simulink model "sampleModel1449_2_sub_sub"  (R2023a)
settings: Solver=VariableStepAuto  StartTime=0.0  StopTime=10.0  RelTol=1e-3
libraries: hdlsllib x6, simulink x1
settings Model: Creator=user1  LastModifiedBy=user1

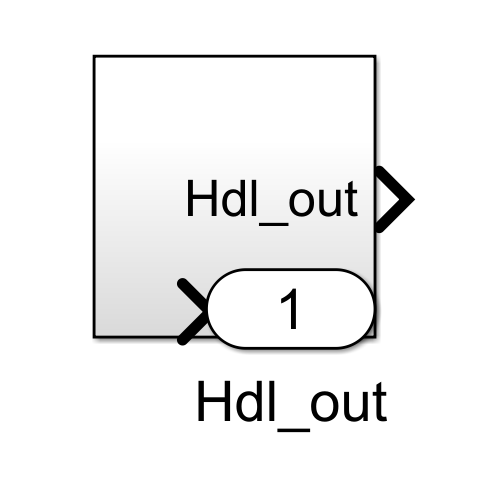
[thumbnail: Simulink's stored preview of the top-level diagram]
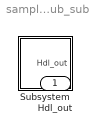
== system sampleModel1449_2_sub_sub ==
  Subsystem : Subsystem
  Hdl_out : Outport  OutDataTypeStr=uint8

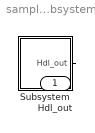
== system sampleModel1449_2_sub_sub/Subsystem ==
  Subsystem : Subsystem
  Hdl_out : Outport  OutDataTypeStr=uint8
  wires:
  Subsystem/1(Hdl_out) -> Hdl_out/1

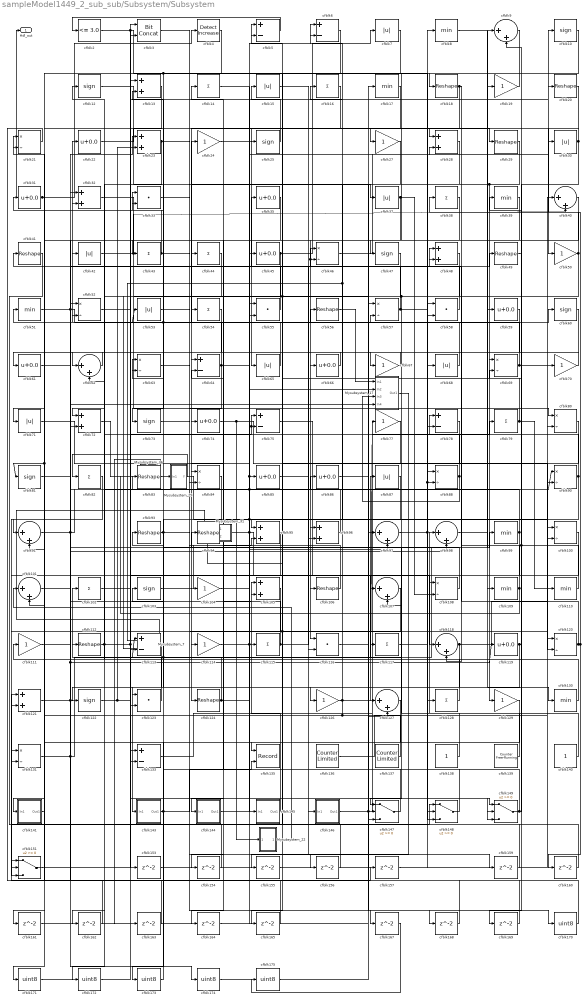
== system sampleModel1449_2_sub_sub/Subsystem/Subsystem ==
  Mysubsystem_17 : Subsystem  TreatAsAtomicUnit=on  RTWFcnName=Mysubsystem_17
      settings: RTWFcnNameOpts=User specified  RTWFileNameOpts=Use function name
  Mysubsystem_22 : Subsystem  TreatAsAtomicUnit=on  RTWFcnName=Mysubsystem_22
      settings: RTWFcnNameOpts=User specified  RTWFileNameOpts=Use function name
  Mysubsystem_29 : Subsystem  TreatAsAtomicUnit=on  RTWFcnName=Mysubsystem_29
      settings: RTWFcnNameOpts=User specified  RTWFileNameOpts=Use function name
  Mysubsystem_31 : Subsystem  TreatAsAtomicUnit=on  RTWFcnName=Mysubsystem_31
      settings: RTWFcnNameOpts=User specified  RTWFileNameOpts=Use function name
  Mysubsystem_36 : Subsystem  TreatAsAtomicUnit=on  RTWFcnName=Mysubsystem_36
      settings: RTWFcnNameOpts=User specified  RTWFileNameOpts=Use function name
  Mysubsystem_7 : Subsystem  TreatAsAtomicUnit=on  RTWFcnName=Mysubsystem_7
      settings: RTWFcnNameOpts=User specified  RTWFileNameOpts=Use function name
  cfblk{10,12,25,47,60,73,81,103,122} (9 alike) : Signum
  cfblk{21,46,52,57,63,69,80,84,88,90,100,108,120,131} (14 alike) : Product  Inputs=*/  OutDataTypeStr=uint8  RndMeth=Zero  SaturateOnIntegerOverflow=on
  cfblk{9,40,62,91,97..98,101,107,118,127} (10 alike) : Sum  Inputs=|++  OutDataTypeStr=uint8
  cfblk{14,16,38,43..44,54,79,82,102,115,117,128} (12 alike) : Sum  Inputs=+  OutDataTypeStr=uint8
  cfblk{19,24,27,50,67,70,77,104,111,114,126,129} (12 alike) : Gain  OutDataTypeStr=uint8
  cfblk{13,23,28,32,48,72,95..96,105,121} (10 alike) : Sum  OutDataTypeStr=uint8
  cfblk{18,20,29,41,49,56,83,93..94,106,112,124} (12 alike) : Reshape
  cfblk{8,17,39,51,99,109..110,130} (8 alike) : MinMax  OutDataTypeStr=uint8
  cfblk{5..6,64,75,78,113,133} (7 alike) : Sum  Inputs=+-  OutDataTypeStr=uint8
  cfblk{33,55,58,116,123} (5 alike) : DotProduct  OutDataTypeStr=uint8
  cfblk{22,31,35,45,59,61,66,74,85..86,119} (11 alike) : Bias  Bias=0.0  SaturateOnIntegerOverflow=off
  cfblk135 : Record  FileSettingsInternal="{\"entries\":[{\"content\":{\"excelSettings\":{\"content\":{},\"type\":\"Streamout.ExcelSettings\"}},\"type\":\"Streamout.FileSettingStorage\",\"uuid\":\"\"}],\"packageUris\":[\"http:\\/\\/schema.mathworks.com\\/mf0\\/streamout_blocks\\/R2020a\"],\"version\":\"1.0\"}"  Layout=[1 1]  SignalsInternal="{\"entries\":[{\"content\":{\"signals\":[{\"content\":{\"blockPath\":[],\"dimensions\":[1],\"domain\":\"\",\"lineColor\":\"#a2142f\",\"plots\":[1],\"port\":1,\"signalID\":18032,\"signalName\":\"cfblk48\"},\"type\":\"RecordBlkView.Signal\",\"uuid\":\"\"},{\"content\":{\"blockPath\":[],\"dimensions\":[1],\"domain\":\"\",\"lineColor\":\"#139fff\",\"plots\":[1],\"port\":2,\"signalID\":18035,\"signalName\":\"cfblk143\"},\"type\":\"RecordBlkView.Signal\",\"uuid\":\"\"}]},\"type\":\"RecordBlkView.InputSignals\",\"uuid\":\"\"}],\"packageUris\":[\"http:\\/\\/schema.mathworks.com\\/mf0\\/streamout_blocks\\/R2020a\"],\"version\":\"1.0\"}"  VisualizationBindings="{\"xyplotplugin\":{\"info\":[{\"series\":[{\"bindingParametersList\":[{\"parameter\":\"X-Axis\",\"signalID\":18032,\"signalName\":\"cfblk48\"},{\"parameter\":\"Y-Axis\",\"signalID\":18035,\"signalName\":\"cfblk143\"}],\"seriesID\":15856}],\"subplotID\":1}]}}"  CompatibilityTag=XY  st=-1
  cfblk136 : hdlsllib/Sources/Counter Limited  uplimit=7  tsamp=-1
  cfblk137 : hdlsllib/Sources/Counter Limited  uplimit=7  tsamp=-1
  cfblk138 : Constant  OutDataTypeStr=uint8  SampleTime=-1
  cfblk139 : hdlsllib/Sources/Counter Free-Running  NumBits=16  tsamp=-1
  cfblk140 : Constant  OutDataTypeStr=uint8  SampleTime=-1
  cfblk141 : Subsystem
      settings: LibrarySourceBlock=|
      | hdlsllib/Ports &
      | Subsystems/Subsystem
  cfblk143 : Subsystem
      settings: LibrarySourceBlock=|
      | hdlsllib/Ports &
      | Subsystems/Subsystem
  cfblk144 : Subsystem
      settings: LibrarySourceBlock=|
      | hdlsllib/Ports &
      | Subsystems/Subsystem
  cfblk145 : Subsystem
      settings: LibrarySourceBlock=|
      | hdlsllib/Ports &
      | Subsystems/Subsystem
  cfblk146 : Subsystem
      settings: LibrarySourceBlock=|
      | hdlsllib/Ports &
      | Subsystems/Subsystem
  cfblk{147..149,151} (4 alike) : Switch  OutDataTypeStr=uint8  SaturateOnIntegerOverflow=off  InputSameDT=off
  cfblk{7,15,30,37,42,53,65,68,71,87} (10 alike) : Abs  OutDataTypeStr=uint8  SaturateOnIntegerOverflow=off
  cfblk{153..157,159..165,167..169} (15 alike) : Delay  SampleTime=1
  cfblk{170..175} (6 alike) : DataTypeConversion  OutDataTypeStr=uint8  SaturateOnIntegerOverflow=off  RndMeth=Floor
  cfblk2 : hdlsllib/Logic and Bit Operations/Compare To Constant  relop=<=  const=3.0  OutDataTypeStr=uint8
  cfblk3 : hdlsllib/Logic and Bit Operations/Bit Concat  numInputs=2
  cfblk4 : simulink/Logic and Bit Operations/Detect Increase  vinit=0.0  OutDataTypeStr=uint8
      settings: LibrarySourceBlock=|
      | hdlsllib/Logic and Bit
      | Operations/Detect
      | Increase
  Hdl_out : Outport  OutDataTypeStr=uint8
  wires:
  Mysubsystem_36/1(Out1) -> cfblk163/1
  cfblk72/1 -> Mysubsystem_36/1(In1)
  Mysubsystem_7/1(Out1) -> Mysubsystem_31/2(In2)
  Mysubsystem_29/1(Y) -> cfblk82/1
  Mysubsystem_22/1(Out1) -> cfblk101/1
  Mysubsystem_17/1(Out1) -> cfblk155/1
  cfblk56/1 -> Mysubsystem_17/1(In1)
  cfblk175/1 -> cfblk127/2
  cfblk167/1 -> cfblk175/1
  cfblk174/1 -> cfblk127/1
  cfblk173/1 -> cfblk103/1
  cfblk127/1 -> cfblk173/1
  cfblk172/1 -> cfblk3/2
  cfblk171/1 -> cfblk3/1
  cfblk129/1 -> cfblk171/1
  cfblk170/1 -> cfblk52/1
  cfblk3/1 -> cfblk170/1
  cfblk169/1 -> cfblk151/2
  cfblk49/1 -> cfblk169/1
  cfblk168/1 -> cfblk121/1
  cfblk86/1 -> cfblk168/1
  cfblk165/1 -> cfblk133/1
  cfblk9/1 -> cfblk165/1
  cfblk164/1 -> cfblk57/1
  cfblk39/1 -> cfblk164/1
  cfblk163/1 -> cfblk91/2
  cfblk162/1 -> cfblk151/1
  cfblk161/1 -> cfblk55/1
  cfblk160/1 -> cfblk5/2
  cfblk159/1 -> cfblk131/1
  cfblk15/1 -> cfblk159/1
  cfblk157/1 -> cfblk100/1
  cfblk21/1 -> cfblk157/1
  cfblk156/1 -> cfblk13/1
  cfblk63/1 -> cfblk156/1
  cfblk155/1 -> cfblk88/1
  cfblk154/1 -> cfblk32/1
  cfblk95/1 -> cfblk154/1
  cfblk153/1 -> cfblk58/2
  cfblk102/1 -> cfblk153/1
  cfblk7/1 -> cfblk101/2, cfblk43/1
  cfblk77/1 -> cfblk96/2
  cfblk148/1 -> cfblk64/2
  cfblk94/1 -> cfblk148/3, cfblk120/2
  cfblk105/1 -> cfblk131/2
  cfblk81/1 -> cfblk23/1
  cfblk136/1 -> cfblk70/1
  cfblk54/1 -> cfblk91/1
  cfblk80/1 -> cfblk148/2
  cfblk65/1 -> cfblk21/1
  cfblk90/1 -> cfblk107/2, cfblk32/2
  cfblk118/1 -> cfblk122/1, cfblk80/2
  cfblk10/1 -> cfblk47/1
  cfblk146/1(Out1) -> cfblk68/1, cfblk149/2
  cfblk30/1 -> cfblk69/1, cfblk28/1
  cfblk53/1 -> cfblk57/2
  cfblk66/1 -> cfblk64/1
  cfblk33/1 -> cfblk78/2
  cfblk69/1 -> cfblk40/1, cfblk42/1
  cfblk103/1 -> cfblk55/2
  cfblk27/1 -> cfblk96/1
  cfblk70/1 -> cfblk67/1
  cfblk122/1 -> cfblk20/1, cfblk23/2
  cfblk79/1 -> cfblk5/1, cfblk110/1
  cfblk96/1 -> cfblk13/2
  cfblk48/1 -> Mysubsystem_7/2(In2), cfblk135/1
  cfblk112/1 -> cfblk75/1, cfblk75/2, cfblk147/3, cfblk172/1
  cfblk111/1 -> cfblk105/2
  cfblk37/1 -> cfblk72/2, cfblk108/2
  cfblk4/1 -> cfblk73/1
  cfblk109/1 -> Mysubsystem_29/1(In1), cfblk41/1
  cfblk52/1 -> cfblk107/1
  cfblk108/1 -> cfblk63/2
  cfblk32/1 -> cfblk97/1
  cfblk84/1 -> cfblk123/1
  cfblk58/1 -> cfblk14/1
  cfblk73/1 -> cfblk117/1
  cfblk44/1 -> cfblk72/1
  cfblk82/1 -> cfblk151/3
  cfblk19/1 -> cfblk18/1
  cfblk14/1 -> cfblk100/2, cfblk108/1
  cfblk75/1 -> cfblk118/1
  cfblk88/1 -> Mysubsystem_17/3(In3), cfblk78/1
  cfblk110/1 -> cfblk46/1, cfblk46/2, cfblk39/1
  cfblk5/1 -> cfblk2/1
  cfblk20/1 -> cfblk50/1
  cfblk60/1 -> cfblk84/1
  cfblk35/1 -> cfblk141/1(In1)
  cfblk115/1 -> cfblk44/1, cfblk49/1
  cfblk71/1 -> cfblk145/1(In1)
  cfblk149/1 -> cfblk63/1, cfblk69/2
  cfblk62/1 -> cfblk61/1
  cfblk99/1 -> cfblk62/2, cfblk133/2
  cfblk107/1 -> Mysubsystem_31/1(In1), cfblk123/2
  cfblk119/1 -> cfblk126/1, cfblk9/2
  cfblk87/1 -> cfblk144/1(In1)
  cfblk40/1 -> Mysubsystem_7/1(In1), cfblk66/1
  cfblk100/1 -> cfblk121/2
  cfblk114/1 -> cfblk56/1, cfblk149/3
  cfblk106/1 -> cfblk54/1
  cfblk97/1 -> cfblk88/2, cfblk30/1, cfblk149/1
  cfblk2/1 -> cfblk128/1, cfblk104/1
  cfblk91/1 -> cfblk19/1, cfblk98/2
  cfblk98/1 -> cfblk130/1
  cfblk61/1 -> cfblk48/1
  cfblk12/1 -> cfblk45/1
  cfblk128/1 -> cfblk52/2
  cfblk78/1 -> cfblk95/1
  cfblk147/1 -> cfblk93/1, cfblk113/1
  cfblk104/1 -> cfblk90/1, cfblk6/2
  cfblk101/1 -> cfblk99/1
  cfblk83/1 -> cfblk115/1
  cfblk131/1 -> Mysubsystem_17/4(In4), cfblk87/1
  cfblk93/1 -> cfblk53/1, cfblk33/2, cfblk95/2
  cfblk8/1 -> cfblk109/1
  cfblk143/1(Out1) -> cfblk33/1, cfblk135/2
  cfblk51/1 -> cfblk60/1, cfblk174/1
  cfblk139/1 -> cfblk94/1
  cfblk23/1 -> cfblk37/1, cfblk162/1
  cfblk144/1(Out1) -> cfblk85/1, cfblk28/2
  cfblk47/1 -> cfblk114/1
  cfblk116/1 -> cfblk17/1
  cfblk121/1 -> cfblk86/1, cfblk119/1, cfblk59/1
  cfblk126/1 -> cfblk77/1, cfblk16/1
  cfblk6/1 -> cfblk81/1, cfblk161/1
  cfblk85/1 -> cfblk146/1(In1)
  cfblk140/1 -> cfblk98/1
  cfblk137/1 -> cfblk6/1, cfblk21/2
  cfblk57/1 -> cfblk35/1, cfblk90/2
  cfblk17/1 -> cfblk25/1
  cfblk28/1 -> cfblk74/1
  cfblk133/1 -> cfblk79/1
  cfblk13/1 -> cfblk71/1
  cfblk25/1 -> cfblk15/1
  cfblk29/1 -> cfblk129/1, cfblk147/2
  cfblk113/1 -> cfblk143/1(In1)
  cfblk59/1 -> cfblk106/1
  cfblk50/1 -> cfblk147/1, cfblk116/2, cfblk10/1
  cfblk117/1 -> cfblk8/1
  cfblk55/1 -> cfblk12/1
  cfblk68/1 -> cfblk22/1
  cfblk151/1 -> cfblk58/1
  cfblk145/1(Out1) -> cfblk105/1
  cfblk64/1 -> Mysubsystem_17/2(In2), cfblk24/1, cfblk84/2
  cfblk141/1(Out1) -> cfblk51/1
  cfblk46/1 -> cfblk9/1
  cfblk130/1 -> cfblk111/1
  cfblk16/1 -> cfblk124/1
  cfblk31/1 -> cfblk4/1, Hdl_out/1
  cfblk38/1 -> cfblk116/1
  cfblk41/1 -> cfblk148/1
  cfblk24/1 -> cfblk65/1
  cfblk138/1 -> cfblk112/1
  cfblk120/1 -> cfblk38/1, cfblk160/1, cfblk48/2
  cfblk22/1 -> cfblk29/1
  cfblk18/1 -> cfblk27/1, cfblk118/2
  cfblk124/1 -> cfblk83/1, cfblk97/2
  cfblk123/1 -> cfblk102/1
  cfblk43/1 -> cfblk31/1, cfblk167/1
  cfblk67/1 -> cfblk62/1
  cfblk74/1 -> Mysubsystem_22/1(In1), cfblk120/1
  cfblk42/1 -> cfblk80/1, cfblk40/2
  cfblk45/1 -> cfblk7/1, cfblk113/2

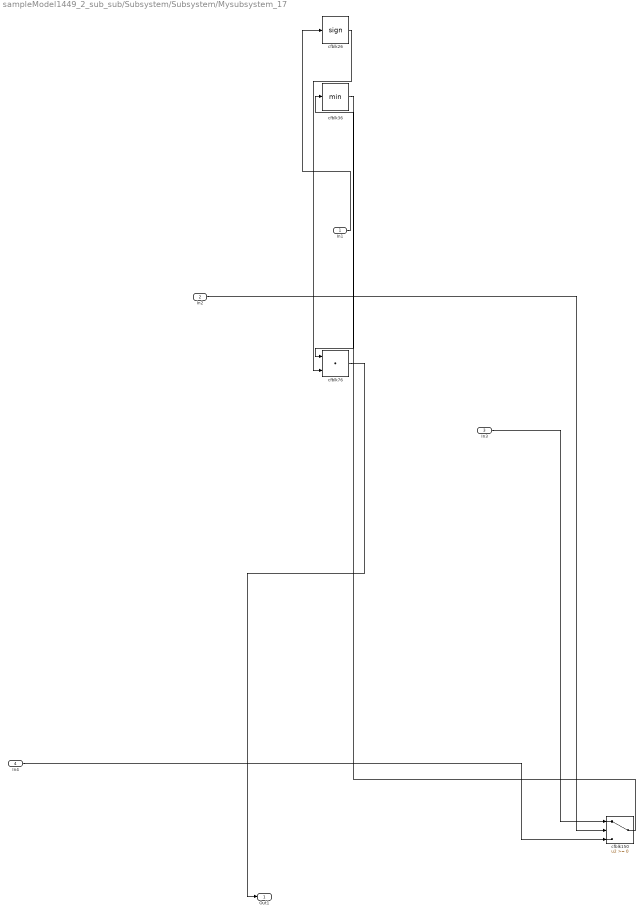
== system sampleModel1449_2_sub_sub/Subsystem/Subsystem/Mysubsystem_17 ==
  In1 : Inport
  In2 : Inport  Port=2
  In3 : Inport  Port=3
  In4 : Inport  Port=4
  cfblk150 : Switch  SaturateOnIntegerOverflow=off  InputSameDT=off
  cfblk26 : Signum
  cfblk36 : MinMax
  cfblk76 : DotProduct  OutDataTypeStr=Inherit: Inherit via internal rule
  Out1 : Outport
  wires:
  cfblk76/1 -> Out1/1
  cfblk26/1 -> cfblk76/2
  cfblk150/1 -> cfblk36/1
  cfblk36/1 -> cfblk76/1
  In4/1 -> cfblk150/3
  In1/1 -> cfblk26/1
  In3/1 -> cfblk150/1
  In2/1 -> cfblk150/2

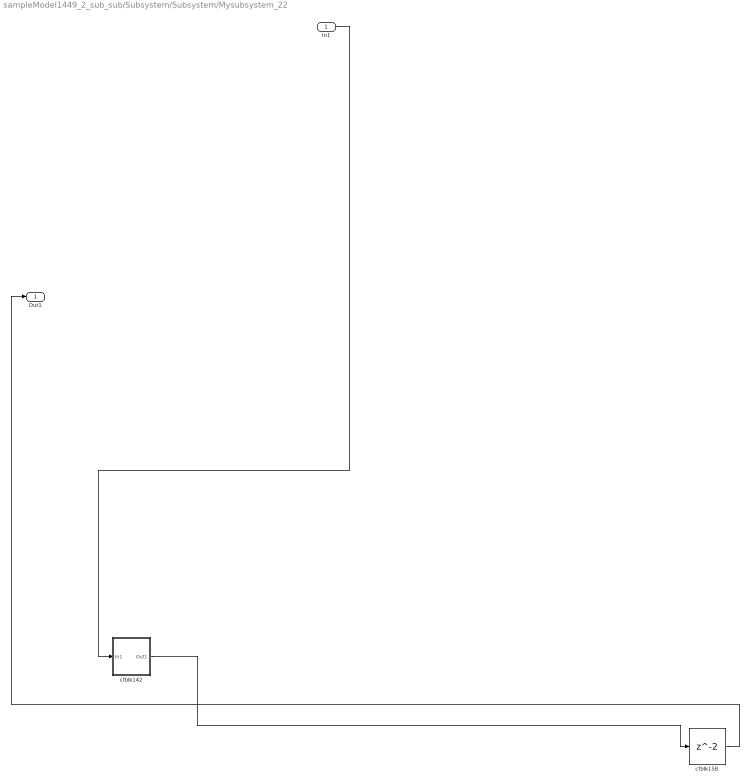
== system sampleModel1449_2_sub_sub/Subsystem/Subsystem/Mysubsystem_22 ==
  In1 : Inport
  cfblk142 : Subsystem
      settings: LibrarySourceBlock=|
      | hdlsllib/Ports &
      | Subsystems/Subsystem
  cfblk158 : Delay  SampleTime=1
  Out1 : Outport
  wires:
  cfblk142/1(Out1) -> cfblk158/1
  In1/1 -> cfblk142/1(In1)
  cfblk158/1 -> Out1/1

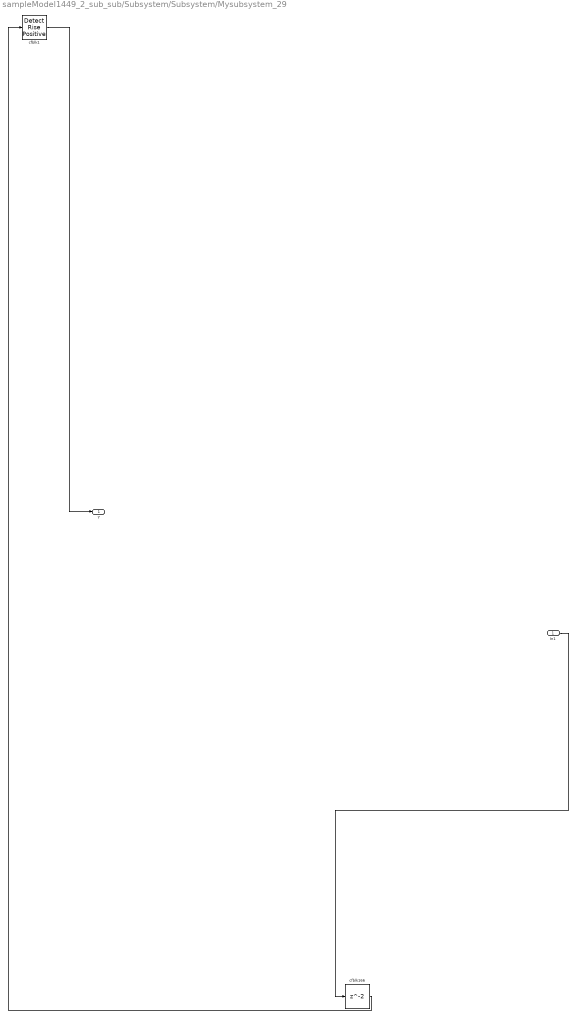
== system sampleModel1449_2_sub_sub/Subsystem/Subsystem/Mysubsystem_29 ==
  In1 : Inport
  cfblk1 : hdlsllib/Logic and Bit Operations/Detect Rise Positive  vinit=0  OutDataTypeStr=boolean
  cfblk166 : Delay  SampleTime=1
  Y : Outport
  wires:
  cfblk166/1 -> cfblk1/1
  cfblk1/1 -> Y/1
  In1/1 -> cfblk166/1

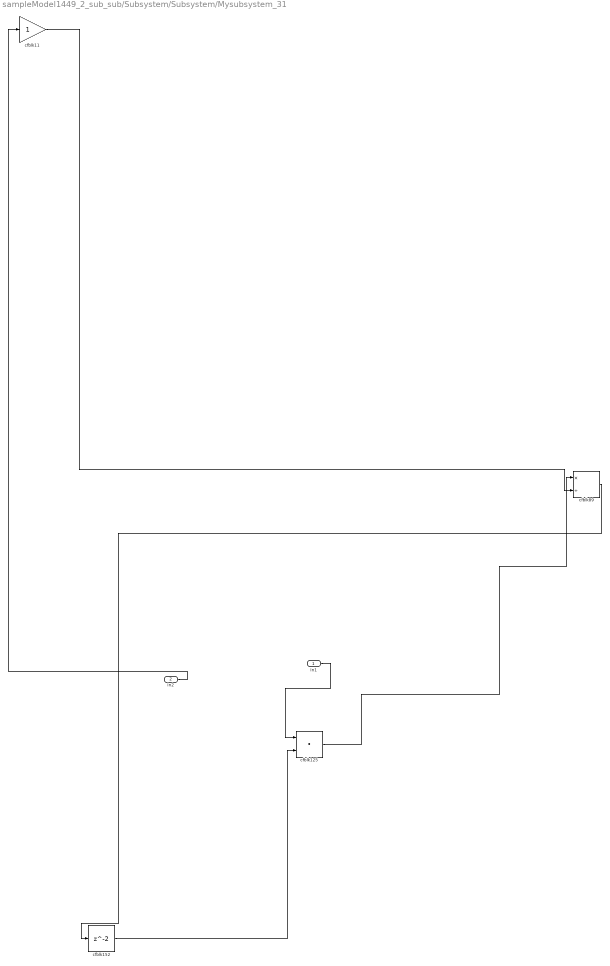
== system sampleModel1449_2_sub_sub/Subsystem/Subsystem/Mysubsystem_31 ==
  In1 : Inport
  In2 : Inport  Port=2
  cfblk11 : Gain
  cfblk125 : DotProduct  OutDataTypeStr=Inherit: Inherit via internal rule
  cfblk152 : Delay  SampleTime=1
  cfblk89 : Product  Inputs=*/  RndMeth=Zero  SaturateOnIntegerOverflow=on
  wires:
  cfblk152/1 -> cfblk125/2
  cfblk89/1 -> cfblk152/1
  cfblk125/1 -> cfblk89/1
  In2/1 -> cfblk11/1
  cfblk11/1 -> cfblk89/2
  In1/1 -> cfblk125/1

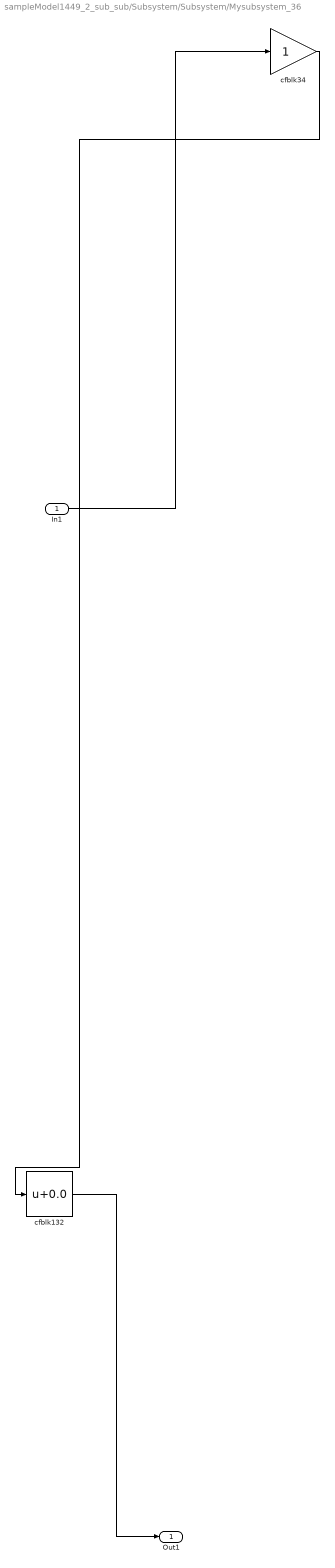
== system sampleModel1449_2_sub_sub/Subsystem/Subsystem/Mysubsystem_36 ==
  In1 : Inport
  cfblk132 : Bias  Bias=0.0  SaturateOnIntegerOverflow=off
  cfblk34 : Gain
  Out1 : Outport
  wires:
  cfblk34/1 -> cfblk132/1
  In1/1 -> cfblk34/1
  cfblk132/1 -> Out1/1

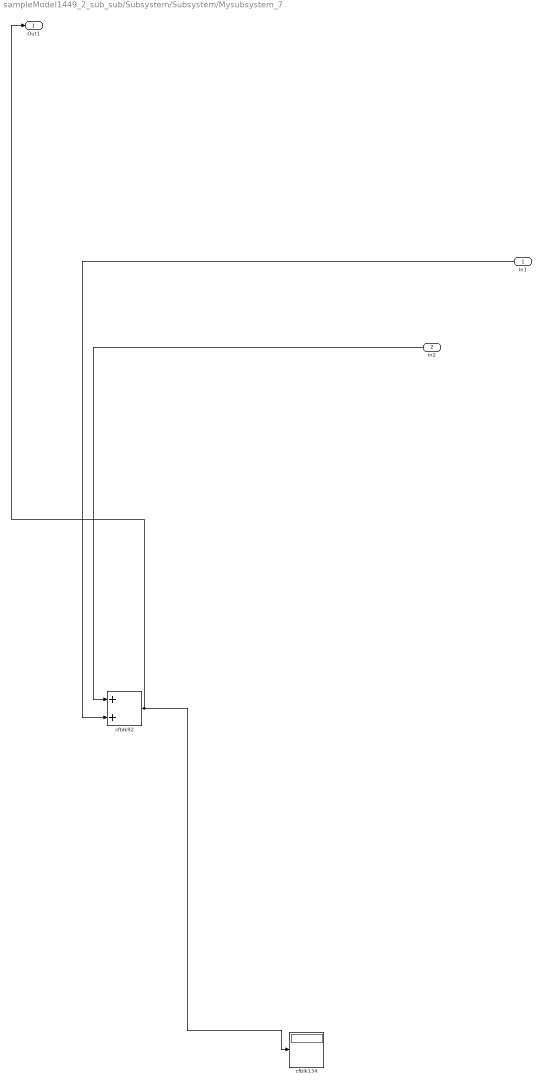
== system sampleModel1449_2_sub_sub/Subsystem/Subsystem/Mysubsystem_7 ==
  In1 : Inport
  In2 : Inport  Port=2
  cfblk134 : Display
  cfblk92 : Sum
  Out1 : Outport
  wires:
  cfblk92/1 -> Out1/1, cfblk134/1
  In2/1 -> cfblk92/1
  In1/1 -> cfblk92/2

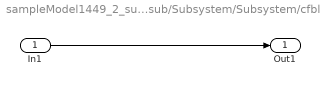
== system sampleModel1449_2_sub_sub/Subsystem/Subsystem/cfblk141 ==
  In1 : Inport
  Out1 : Outport
  wires:
  In1/1 -> Out1/1

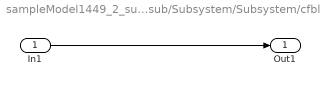
== system sampleModel1449_2_sub_sub/Subsystem/Subsystem/cfblk143 ==
  In1 : Inport
  Out1 : Outport
  wires:
  In1/1 -> Out1/1

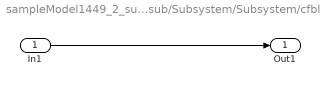
== system sampleModel1449_2_sub_sub/Subsystem/Subsystem/cfblk144 ==
  In1 : Inport
  Out1 : Outport
  wires:
  In1/1 -> Out1/1

== system sampleModel1449_2_sub_sub/Subsystem/Subsystem/cfblk145 ==
  In1 : Inport
  Out1 : Outport
  wires:
  In1/1 -> Out1/1

== system sampleModel1449_2_sub_sub/Subsystem/Subsystem/cfblk146 ==
  In1 : Inport
  Out1 : Outport
  wires:
  In1/1 -> Out1/1

== system sampleModel1449_2_sub_sub/Subsystem/Subsystem/Mysubsystem_22/cfblk142 ==
  In1 : Inport
  Out1 : Outport
  wires:
  In1/1 -> Out1/1
